simulink model "lab5part2"  (R2025b)
settings: Solver=ode3  StartTime=0.0  StopTime=5000  RelTol=1e-3
libraries: dspsrcs4 x1
settings Model: Creator=hvc2260  LastModifiedBy=hvc2260

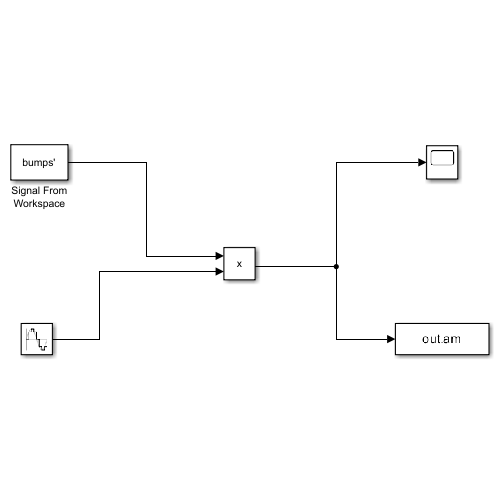
[thumbnail: Simulink's stored preview of the top-level diagram]
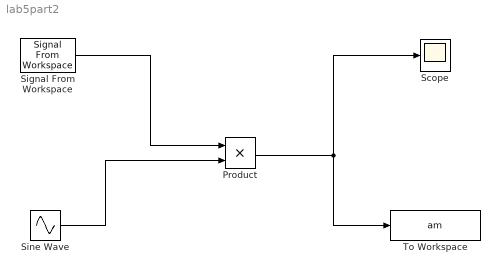
== system lab5part2 ==
  Product : Product
  Scope : Scope
      settings: ActiveDisplayYMinimum=-1  ActiveDisplayYMaximum=1
  Signal From Workspace : dspsrcs4/Signal From Workspace  X=bumps'  Ts=1  nsamps=1  OutputAfterFinalValue=Setting to zero  ignoreOrWarnInputAndFrameLengths=off  OutputFrames=off
  Sine Wave : Sin  Frequency=2*pi*0.3  Phase=pi/2  SampleTime=1
  To Workspace : ToWorkspace  VariableName=am  SampleTime=-1
  wires:
  Signal From Workspace/1 -> Product/1
  Sine Wave/1 -> Product/2
  Product/1 -> To Workspace/1, Scope/1
